simulink model "OneDofAeroVTOL_control101_2025b"  (R2025b)
settings: Solver=VariableStepAuto  StartTime=0.0  StopTime=Stoptime  RelTol=1e-3
PreLoadFcn:
  | run("OneDofAeroVTOL_Data_control101.m");
values from neighbouring files (symbols this model uses):
  Bl_P = 0.002    [OneDofAeroVTOL_Data_control101.m]    (also in OneDofAeroVTOL_model_control101.m)
  Bm_P = 0.014293    [FanAndPlate_Data_control101.m]    (also in FanAndPlate_model_control101.m; OneDofAeroVTOL_Data_control101.m = 0.001; OneDofAeroVTOL_model_control101.m = 0.001)
  g_P = 9.81    [FanAndPlate_Data_control101.m]    (also in FanAndPlate_model_control101.m; OneDofAeroVTOL_Data_control101.m; OneDofAeroVTOL_model_control101.m)
  Jl_P = 0.00017    [OneDofAeroVTOL_Data_control101.m]    (also in OneDofAeroVTOL_model_control101.m)
  Jm_P = 0.0000536    (= 5.36e-05)    [FanAndPlate_Data_control101.m]    (also in FanAndPlate_model_control101.m; OneDofAeroVTOL_Data_control101.m = 0.000184; OneDofAeroVTOL_model_control101.m = 0.000184)
  Kb_P = 0.077    [FanAndPlate_Data_control101.m]    (also in FanAndPlate_model_control101.m; OneDofAeroVTOL_Data_control101.m = 0.0577; OneDofAeroVTOL_model_control101.m = 0.0577)
  Kf_P = 0.0002    [OneDofAeroVTOL_Data_control101.m]    (also in OneDofAeroVTOL_model_control101.m)
  Kpl_P = 0.0001    [FanAndPlate_Data_control101.m]    (also in FanAndPlate_model_control101.m; OneDofAeroVTOL_Data_control101.m = 1e-05; OneDofAeroVTOL_model_control101.m = 1e-05)
  Kt_P = 0.077    [FanAndPlate_Data_control101.m]    (also in FanAndPlate_model_control101.m; OneDofAeroVTOL_Data_control101.m = 0.0577; OneDofAeroVTOL_model_control101.m = 0.0577)
  l1_P = 0.0156    [OneDofAeroVTOL_Data_control101.m]    (also in OneDofAeroVTOL_model_control101.m)
  l2_P = 0.0056    [OneDofAeroVTOL_Data_control101.m]    (also in OneDofAeroVTOL_model_control101.m)
  l3_P = 0.0035    [OneDofAeroVTOL_Data_control101.m]    (also in OneDofAeroVTOL_model_control101.m)
  Lm_P = 0.0000177    (= 1.77e-05)    [FanAndPlate_Data_control101.m]    (also in FanAndPlate_model_control101.m; OneDofAeroVTOL_Data_control101.m = 0.00538; OneDofAeroVTOL_model_control101.m = 0.00538)
  m1_P = 0.068    [OneDofAeroVTOL_Data_control101.m]    (also in OneDofAeroVTOL_model_control101.m)
  m2_P = 0.27    [OneDofAeroVTOL_Data_control101.m]    (also in OneDofAeroVTOL_model_control101.m)
  m3_P = 0.048    [OneDofAeroVTOL_Data_control101.m]    (also in OneDofAeroVTOL_model_control101.m)
  Rm_P = 0.0305    [FanAndPlate_Data_control101.m]    (also in FanAndPlate_model_control101.m; OneDofAeroVTOL_Data_control101.m = 8.4; OneDofAeroVTOL_model_control101.m = 8.4)
undefined symbols (not defined in the file or in its folder): fanspeed, initialcurrent, initialplateangle, initialplatespeed, SampleTime
settings Model: Creator=sword  LastModifiedBy=Anthony Rossiter
settings DebuggingCC: InheritedTsInSrcMsg=none
settings RTWCC: GPUComputeCapability=3.5

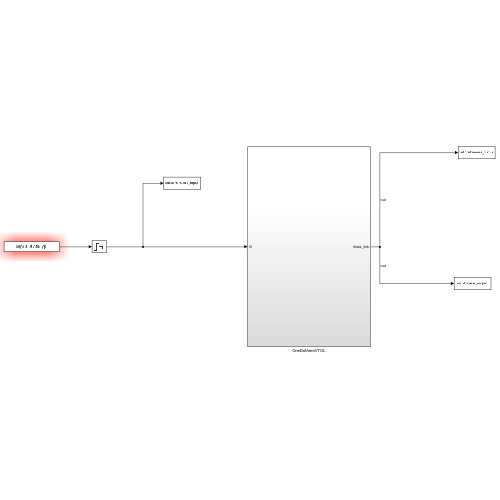
[thumbnail: Simulink's stored preview of the top-level diagram]
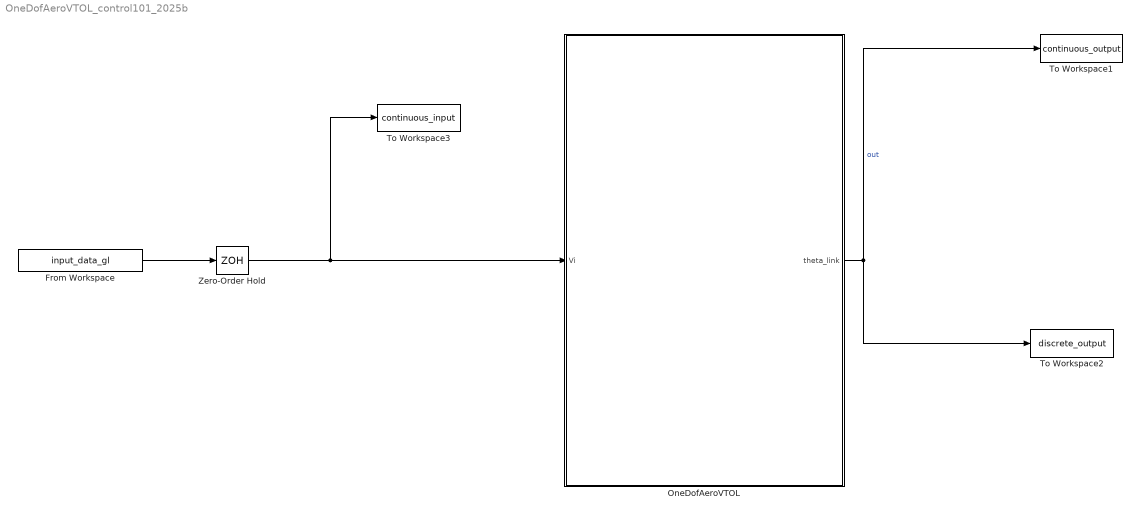
== system OneDofAeroVTOL_control101_2025b ==
  From Workspace : FromWorkspace  VariableName=input_data_gl  SampleTime=SampleTime
  OneDofAeroVTOL : Subsystem
  To Workspace1 : ToWorkspace  VariableName=continuous_output  SaveFormat=Structure With Time  SampleTime=-1
  To Workspace2 : ToWorkspace  VariableName=discrete_output  SaveFormat=Structure With Time  SampleTime=SampleTime
  To Workspace3 : ToWorkspace  VariableName=continuous_input  SaveFormat=Structure With Time  SampleTime=SampleTime
  Zero-Order Hold : ZeroOrderHold  SampleTime=SampleTime
  wires:
  OneDofAeroVTOL/1(theta_link) -> To Workspace1/1, To Workspace2/1  "out"
  From Workspace/1 -> Zero-Order Hold/1
  Zero-Order Hold/1 -> To Workspace3/1, OneDofAeroVTOL/1(Vi)

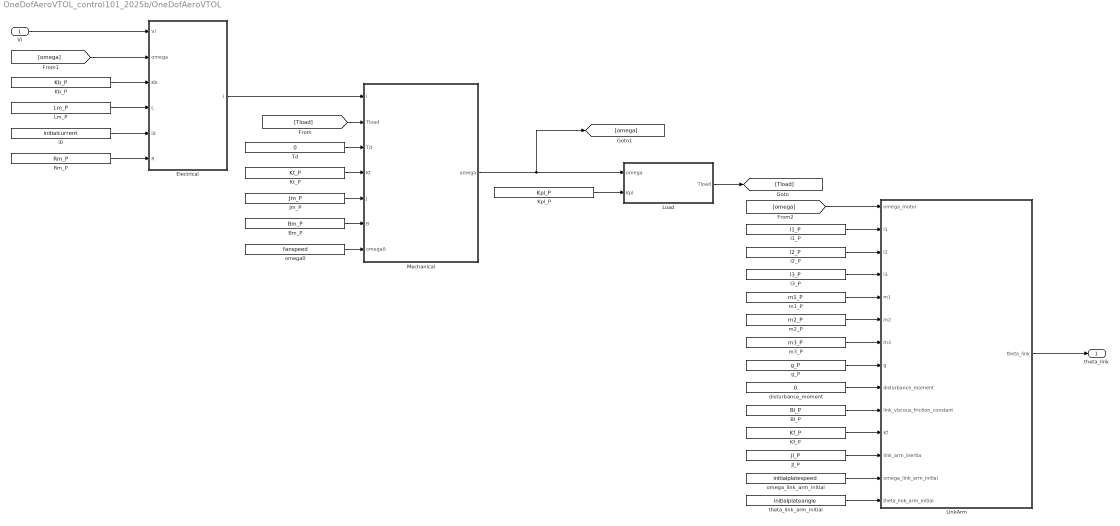
== system OneDofAeroVTOL_control101_2025b/OneDofAeroVTOL ==
  Vi : Inport
  Bl_P : Constant  Value=Bl_P  OutDataTypeStr=Inherit: Inherit via back propagation  SampleTime=-1
  Bm_P : Constant  Value=Bm_P  OutDataTypeStr=Inherit: Inherit via back propagation  SampleTime=-1
  Electrical : Subsystem
  Jl_P : Constant  Value=Jl_P  OutDataTypeStr=Inherit: Inherit via back propagation  SampleTime=-1
  Jm_P : Constant  Value=Jm_P  OutDataTypeStr=Inherit: Inherit via back propagation  SampleTime=-1
  Kb_P : Constant  Value=Kb_P  OutDataTypeStr=Inherit: Inherit via back propagation  SampleTime=-1
  Kf_P : Constant  Value=Kf_P  OutDataTypeStr=Inherit: Inherit via back propagation  SampleTime=-1
  Kpl_P : Constant  Value=Kpl_P  OutDataTypeStr=Inherit: Inherit via back propagation  SampleTime=-1
  Kt_P : Constant  Value=Kt_P  OutDataTypeStr=Inherit: Inherit via back propagation  SampleTime=-1
  LinkArm : Subsystem
  Lm_P : Constant  Value=Lm_P  OutDataTypeStr=Inherit: Inherit via back propagation  SampleTime=-1
  Load : Subsystem
  Mechanical : Subsystem
  Rm_P : Constant  Value=Rm_P  OutDataTypeStr=Inherit: Inherit via back propagation  SampleTime=-1
  Td : Constant  Value=0  OutDataTypeStr=Inherit: Inherit via back propagation  SampleTime=-1
  disturbance_moment : Constant  Value=0  OutDataTypeStr=Inherit: Inherit via back propagation  SampleTime=-1
  g_P : Constant  Value=g_P  OutDataTypeStr=Inherit: Inherit via back propagation  SampleTime=-1
  i0 : Constant  Value=initialcurrent  OutDataTypeStr=Inherit: Inherit via back propagation  SampleTime=-1
  l1_P : Constant  Value=l1_P  OutDataTypeStr=Inherit: Inherit via back propagation  SampleTime=-1
  l2_P : Constant  Value=l2_P  OutDataTypeStr=Inherit: Inherit via back propagation  SampleTime=-1
  l3_P : Constant  Value=l3_P  OutDataTypeStr=Inherit: Inherit via back propagation  SampleTime=-1
  m1_P : Constant  Value=m1_P  OutDataTypeStr=Inherit: Inherit via back propagation  SampleTime=-1
  m2_P : Constant  Value=m2_P  OutDataTypeStr=Inherit: Inherit via back propagation  SampleTime=-1
  m3_P : Constant  Value=m3_P  OutDataTypeStr=Inherit: Inherit via back propagation  SampleTime=-1
  omega0 : Constant  Value=fanspeed  OutDataTypeStr=Inherit: Inherit via back propagation  SampleTime=-1
  omega_link_arm_initial : Constant  Value=initialplatespeed  OutDataTypeStr=Inherit: Inherit via back propagation  SampleTime=-1
  theta_link_arm_initial : Constant  Value=initialplateangle  OutDataTypeStr=Inherit: Inherit via back propagation  SampleTime=-1
  theta_link : Outport  VectorParamsAs1DForOutWhenUnconnected=off
  wires:
  g_P/1 -> LinkArm/8(g)
  theta_link_arm_initial/1 -> LinkArm/14(theta_link_arm_initial)
  LinkArm/1(theta_link) -> theta_link/1
  Bl_P/1 -> LinkArm/10(link_viscous_friction_constant)
  m2_P/1 -> LinkArm/6(m2)
  Jl_P/1 -> LinkArm/12(link_arm_inertia)
  l1_P/1 -> LinkArm/2(l1)
  disturbance_moment/1 -> LinkArm/9(disturbance_moment)
  m1_P/1 -> LinkArm/5(m1)
  omega_link_arm_initial/1 -> LinkArm/13(omega_link_arm_initial)
  Electrical/1(i) -> Mechanical/1(i)
  Mechanical/1(omega) -> [omega], Load/1(omega)
  Vi/1 -> Electrical/1(Vi)
  Load/1(Tload) -> [Tload]
  [Tload] -> Mechanical/2(Tload)
  Td/1 -> Mechanical/3(Td)
  [omega] -> Electrical/2(omega)
  Kb_P/1 -> Electrical/3(Kb)
  i0/1 -> Electrical/5(i0)
  Lm_P/1 -> Electrical/4(L)
  Rm_P/1 -> Electrical/6(R)
  Kpl_P/1 -> Load/2(Kpl)
  Kt_P/1 -> Mechanical/4(Kt)
  Jm_P/1 -> Mechanical/5(J)
  Bm_P/1 -> Mechanical/6(B)
  omega0/1 -> Mechanical/7(omega0)
  l2_P/1 -> LinkArm/3(l2)
  l3_P/1 -> LinkArm/4(l3)
  [omega] -> LinkArm/1(omega_motor)
  m3_P/1 -> LinkArm/7(m3)
  Kf_P/1 -> LinkArm/11(Kf)

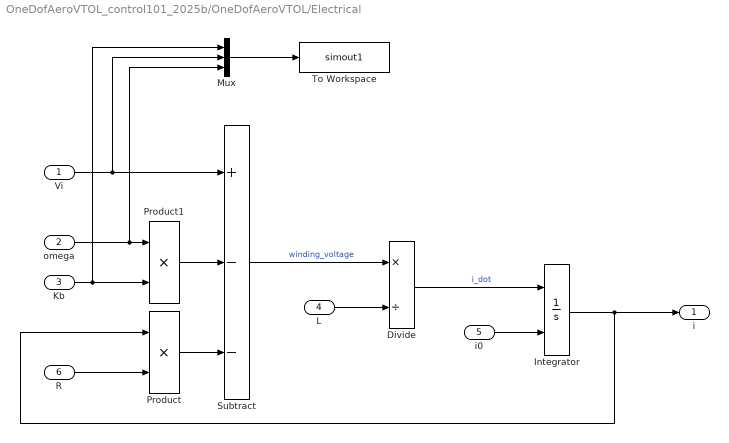
== system OneDofAeroVTOL_control101_2025b/OneDofAeroVTOL/Electrical ==
  Vi : Inport
  omega : Inport  Port=2
  Kb : Inport  Port=3
  L : Inport  Port=4
  i0 : Inport  Port=5
  R : Inport  Port=6
  Divide : Product  Inputs=*/  RndMeth=Zero  SaturateOnIntegerOverflow=on  OutDataTypeStr=Inherit: Same as first input
  Integrator : Integrator  InitialConditionSource=external  ContinuousStateAttributes='current'
  Mux : Mux  Inputs=3
  Product : Product  InputSameDT=on  RndMeth=Zero  SaturateOnIntegerOverflow=on  OutDataTypeStr=Inherit: Same as first input
  Product1 : Product  InputSameDT=on  RndMeth=Zero  SaturateOnIntegerOverflow=on  OutDataTypeStr=Inherit: Same as first input
  Subtract : Sum  Inputs=+--  InputSameDT=on  RndMeth=Zero  SaturateOnIntegerOverflow=on
  To Workspace : ToWorkspace  VariableName=simout1  SaveFormat=Timeseries  SampleTime=-1
  i : Outport
  wires:
  Kb/1 -> Mux/1, Product1/2
  omega/1 -> Mux/3, Product1/1
  Product1/1 -> Subtract/2
  R/1 -> Product/2
  Product/1 -> Subtract/3
  Integrator/1 -> i/1, Product/1
  i0/1 -> Integrator/2
  Divide/1 -> Integrator/1  "i_dot"
  L/1 -> Divide/2
  Subtract/1 -> Divide/1  "winding_voltage"
  Vi/1 -> Mux/2, Subtract/1
  Mux/1 -> To Workspace/1

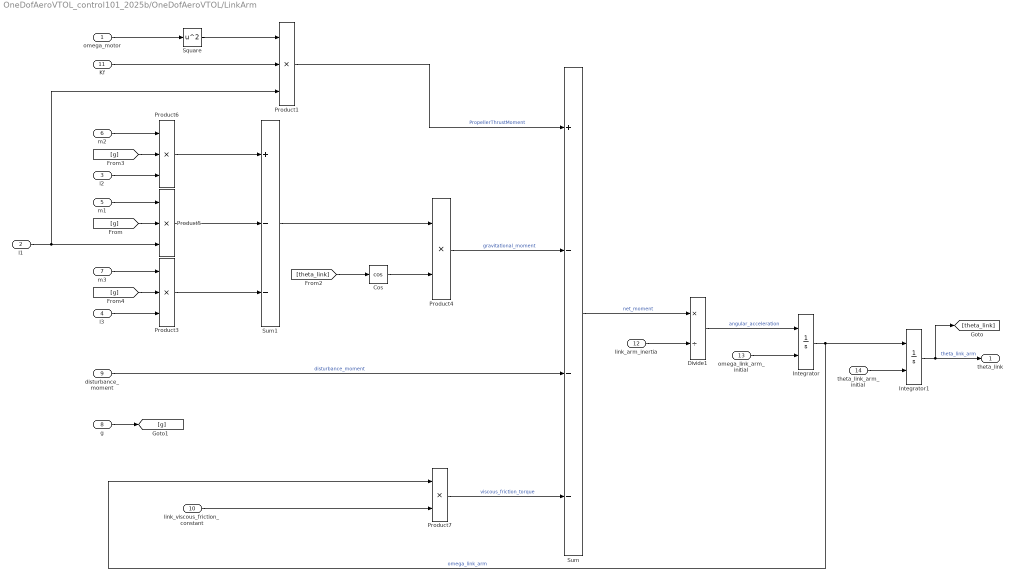
== system OneDofAeroVTOL_control101_2025b/OneDofAeroVTOL/LinkArm ==
  omega_motor : Inport
  l1 : Inport  Port=2
  l2 : Inport  Port=3
  l3 : Inport  Port=4
  m1 : Inport  Port=5
  m2 : Inport  Port=6
  m3 : Inport  Port=7
  g : Inport  Port=8
  disturbance_moment : Inport  Port=9
  link_viscous_friction_constant : Inport  Port=10
  Kf : Inport  Port=11
  link_arm_inertia : Inport  Port=12
  omega_link_arm_initial : Inport  Port=13
  theta_link_arm_initial : Inport  Port=14
  Cos : Trigonometry  Operator=cos
  Divide1 : Product  Inputs=*/  RndMeth=Zero  SaturateOnIntegerOverflow=on  OutDataTypeStr=Inherit: Same as first input
  Integrator : Integrator  InitialConditionSource=external  ContinuousStateAttributes='omega_plate'
  Integrator1 : Integrator  InitialConditionSource=external  ContinuousStateAttributes='theta_plate'
  Product{1,3,5..6} (4 alike) : Product  Inputs=3  InputSameDT=on  RndMeth=Zero  SaturateOnIntegerOverflow=on  OutDataTypeStr=Inherit: Same as first input
  Product4 : Product  InputSameDT=on  RndMeth=Zero  SaturateOnIntegerOverflow=on  OutDataTypeStr=Inherit: Same as first input
  Product7 : Product  InputSameDT=on  RndMeth=Zero  SaturateOnIntegerOverflow=on  OutDataTypeStr=Inherit: Same as first input
  Square : Math  Operator=square
  Sum : Sum  Inputs=+---  OutDataTypeStr=Inherit: Inherit via back propagation  InputSameDT=on  RndMeth=Zero  SaturateOnIntegerOverflow=on
  Sum1 : Sum  Inputs=+--  OutDataTypeStr=Inherit: Inherit via back propagation  InputSameDT=on  RndMeth=Zero  SaturateOnIntegerOverflow=on
  theta_link : Outport
  wires:
  [theta_link] -> Cos/1
  Product1/1 -> Sum/1  "PropellerThrustMoment"
  Sum1/1 -> Product4/1
  Cos/1 -> Product4/2
  Product4/1 -> Sum/2  "gravitational_moment"
  disturbance_moment/1 -> Sum/3  "disturbance_moment"
  Product7/1 -> Sum/4  "viscous_friction_torque"
  link_viscous_friction_constant/1 -> Product7/2
  Sum/1 -> Divide1/1  "net_moment"
  link_arm_inertia/1 -> Divide1/2
  Divide1/1 -> Integrator/1  "angular_acceleration"
  omega_link_arm_initial/1 -> Integrator/2
  Integrator1/1 -> [theta_link], theta_link/1  "theta_link_arm"
  Integrator/1 -> Integrator1/1, Product7/1  "omega_link_arm"
  theta_link_arm_initial/1 -> Integrator1/2
  m1/1 -> Product5/1
  g/1 -> [g]
  [g] -> Product5/2
  l1/1 -> Product5/3, Product1/3
  [g] -> Product6/2
  Product5/1 -> Sum1/2
  Product6/1 -> Sum1/1
  m2/1 -> Product6/1
  l2/1 -> Product6/3
  [g] -> Product3/2
  Product3/1 -> Sum1/3
  m3/1 -> Product3/1
  l3/1 -> Product3/3
  omega_motor/1 -> Square/1
  Square/1 -> Product1/1
  Kf/1 -> Product1/2

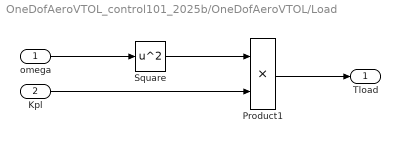
== system OneDofAeroVTOL_control101_2025b/OneDofAeroVTOL/Load ==
  omega : Inport
  Kpl : Inport  Port=2
  Product1 : Product  InputSameDT=on  RndMeth=Zero  SaturateOnIntegerOverflow=on  OutDataTypeStr=Inherit: Same as first input
  Square : Math  Operator=square
  Tload : Outport
  wires:
  Product1/1 -> Tload/1
  Kpl/1 -> Product1/2
  Square/1 -> Product1/1
  omega/1 -> Square/1

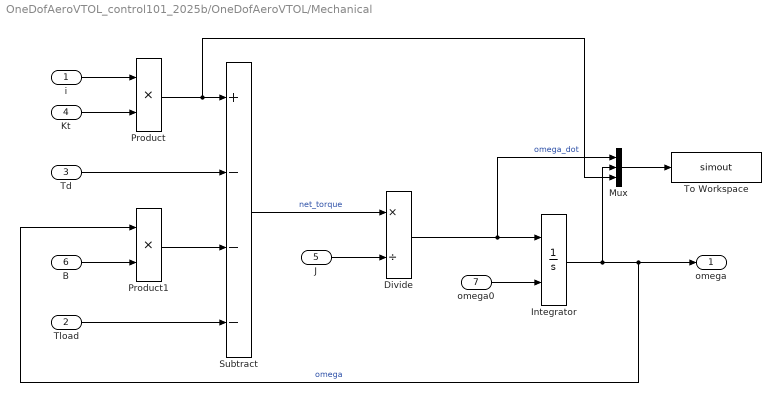
== system OneDofAeroVTOL_control101_2025b/OneDofAeroVTOL/Mechanical ==
  i : Inport
  Tload : Inport  Port=2
  Td : Inport  Port=3
  Kt : Inport  Port=4
  J : Inport  Port=5
  B : Inport  Port=6
  omega0 : Inport  Port=7
  Divide : Product  Inputs=*/  RndMeth=Zero  SaturateOnIntegerOverflow=on  OutDataTypeStr=Inherit: Same as first input
  Integrator : Integrator  InitialConditionSource=external  ContinuousStateAttributes='motor_speed'
  Mux : Mux  Inputs=3
  Product : Product  InputSameDT=on  RndMeth=Zero  SaturateOnIntegerOverflow=on  OutDataTypeStr=Inherit: Same as first input
  Product1 : Product  InputSameDT=on  RndMeth=Zero  SaturateOnIntegerOverflow=on  OutDataTypeStr=Inherit: Same as first input
  Subtract : Sum  Inputs=+---  InputSameDT=on  RndMeth=Zero  SaturateOnIntegerOverflow=on
  To Workspace : ToWorkspace  VariableName=simout  SaveFormat=Timeseries  SampleTime=-1
  omega : Outport
  wires:
  Tload/1 -> Subtract/4
  Td/1 -> Subtract/2
  B/1 -> Product1/2
  Product1/1 -> Subtract/3
  Integrator/1 -> Mux/2, Product1/1, omega/1  "omega"
  Subtract/1 -> Divide/1  "net_torque"
  Divide/1 -> Mux/1, Integrator/1  "omega_dot"
  omega0/1 -> Integrator/2
  J/1 -> Divide/2
  Product/1 -> Mux/3, Subtract/1
  Kt/1 -> Product/2
  i/1 -> Product/1
  Mux/1 -> To Workspace/1
